simulink model "acquire_data_ag"  (R2017b)
settings: Solver=FixedStepDiscrete  StartTime=0.0  StopTime=10.0  RelTol=1e-3
undefined symbols (not defined in the file or in its folder): RGBLED_COLOR_ENUM, RGBLED_MODE_ENUM
libraries: pixhawk_slib_sensors_actuators x3
settings Model: Creator=Mr Wang  LastModifiedBy=dream
settings OptimizationCC: DefaultParameterBehavior=Inlined  MaxStackSize=128
settings DebuggingCC: ParameterTunabilityLossMsg=error
settings HardwareCC: ProdBitPerPointer=32  ProdBitPerSizeT=32  ProdBitPerPtrDiffT=32  ProdLargestAtomicInteger=Long  ProdLargestAtomicFloat=Double  ProdWordSize=32  ProdHWDeviceType=ARM Compatible->ARM Cortex
settings SFSimCC: MATLABDynamicMemAlloc=off
settings RTWCC: SystemTargetFile=ert.tlc  HardwareBoard=Pixhawk PX4  TemplateMakefile=ert_default_tmf  GenerateReport=on  Toolchain=Pixhawk Toolchain  IncludeHyperlinkInReport=on  LaunchReport=on  GenerateTraceInfo=on  GenerateTraceReport=on  GenerateTraceReportSl=on  GenerateTraceReportSf=on  GenerateTraceReportEml=on
settings CodeAppCC: ForceParamTrailComments=on  IgnoreCustomStorageClasses=off  OperatorAnnotations=on  SimulinkDataObjDesc=on  SFDataObjDesc=on  MATLABFcnDesc=on  InsertBlockDesc=on  StateflowObjectComments=on  MATLABSourceComments=on
settings ERTTargetCC: MultiwordLength=2048  ERTCustomFileTemplate=PX4_codertarget_file_process.tlc

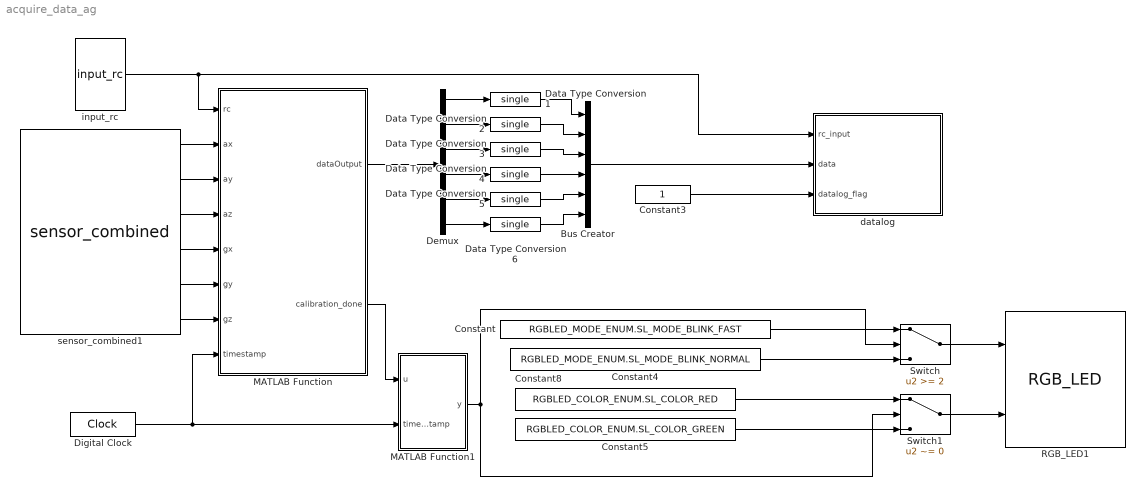
== system acquire_data_ag ==
  Bus Creator : BusCreator  Inputs=6
  Constant : Constant  Value=RGBLED_MODE_ENUM.SL_MODE_BLINK_FAST  OutDataTypeStr=Enum: RGBLED_MODE_ENUM
  Constant3 : Constant  OutDataTypeStr=double
  Constant4 : Constant  Value=RGBLED_MODE_ENUM.SL_MODE_BLINK_NORMAL  OutDataTypeStr=Enum: RGBLED_MODE_ENUM
  Constant5 : Constant  Value=RGBLED_COLOR_ENUM.SL_COLOR_GREEN  OutDataTypeStr=Enum: RGBLED_COLOR_ENUM
  Constant8 : Constant  Value=RGBLED_COLOR_ENUM.SL_COLOR_RED  OutDataTypeStr=Enum: RGBLED_COLOR_ENUM
  Data Type Conversion{1..6} (6 alike) : DataTypeConversion  OutDataTypeStr=single
  Demux : Demux  Outputs=6
  Digital Clock : DigitalClock
  MATLAB Function : MATLAB Function  TreatAsAtomicUnit=on
  MATLAB Function1 : MATLAB Function  TreatAsAtomicUnit=on
  RGB_LED1 : pixhawk_slib_sensors_actuators/RGB_LED  Description=|
      | This block gives the user control over various lighting modes of the RGB LED available on the PX4 hardware. 
      | This block accepts 2 inputs: Mode and Color.  These are enumeration data types.  You can find out what values are valid in the MATLAB command window by typing: 
      | Enumeration members for class 'RGBLED_COLOR_ENUM':
      |     SL_COLOR_OFF
      |     SL_COLOR_RED
      |     SL_COLOR_GREEN
      |     SL_COLOR_BLUE
      |     SL_COLOR_YELLOW
      |     SL_COLOR_PURPLE
      |     SL_COLOR_AMBER
      |     SL_COLOR_CYAN
      |     SL_COLOR_WHITE 
      | Enumeration members for class 'RGBLED_MODE_ENUM':
      |     SL_MODE_OFF
      |     SL_MODE_ON
      |     SL_MODE_DISABLED
      |     SL_MODE_BLINK_SLOW
      |     SL_MODE_BLINK_NORMAL
      |     SL_MODE_BLINK_FAST
      |     SL_MODE_BREATHE  
      | Look at the sample Simulink model: px4demo_rgbled.slx for an example of how to use this block.
      settings: SourceProductName=Pixhawk Target Blocks
  Switch : Switch  Threshold=2
  Switch1 : Switch  Criteria=u2 ~= 0  Threshold=1500
  datalog : Subsystem
  input_rc : pixhawk_slib_sensors_actuators/input_rc  sampletime=1/250  channel1=off  channel2=off  channel3=off  channel4=off  channel5=on  channel6=off  channel7=off  channel8=off  channel9=off  channel10=off  channel11=off  channel12=off  channel13=off  channel14=off  channel15=off  channel16=off  channel17=off  channel18=off  ch_count=off  rssi=off  rc_failsafe=off  rc_lost=off  rc_inputsource=off
      settings: SourceProductName=Pixhawk Target Blocks
  sensor_combined1 : pixhawk_slib_sensors_actuators/sensor_combined  Description=|  sampletime=1/250  show_mag=off  show_acc=on  show_gyro=on  show_baro=off  show_ts=off
      | Sensor Combined Block
      | 
      | This block enables access to the various sensors available on the px4fmu-v2 hardware.  
      | The user can use these signals in the Simulink control model.  
      | The sample time needs to be provided in the mask dialog.  
      | Optional output ports can also be selected.  
      | Refer to the sample model: px4demo_attitude_control.slx
      | 
      | Signal definitions: 
      | Magnetometer (x,y,z) - single values – Magnetic field in NED body frame, in Gauss 
      | Accelerometer (x,y,z) - single values – Acceleration in NED body frame, in m/s^2 
      | Gyroscope (p,q,r) - single values – Angular velocity in radians per second 
      | Barometer (Altitude) - single value – Barometric pressure, already temperature compensated (millibars) 
      | RunTime (timestamp) - double value – Timestamp in microseconds since boot, from gyro 
      |   
      | The sensor_combined block needs to have the px4io service running on the PX4 hardware in order to get valid signal values.
      settings: SourceProductName=Pixhawk Target Blocks
  wires:
  input_rc/1 -> datalog/1(rc_input), MATLAB Function/1(rc)
  Data Type Conversion1/1 -> Bus Creator/1
  Data Type Conversion2/1 -> Bus Creator/2
  Data Type Conversion3/1 -> Bus Creator/3
  Bus Creator/1 -> datalog/2(data)
  MATLAB Function/1(dataOutput) -> Demux/1
  Demux/2 -> Data Type Conversion2/1
  MATLAB Function/2(calibration_done) -> MATLAB Function1/1(u)
  Constant/1 -> Switch/1
  Constant4/1 -> Switch/3
  Switch/1 -> RGB_LED1/1
  Switch1/1 -> RGB_LED1/2
  Constant8/1 -> Switch1/1
  Constant5/1 -> Switch1/3
  Demux/1 -> Data Type Conversion1/1
  Demux/3 -> Data Type Conversion3/1
  Constant3/1 -> datalog/3(datalog_flag)
  Demux/6 -> Data Type Conversion6/1
  Data Type Conversion6/1 -> Bus Creator/6
  Demux/5 -> Data Type Conversion5/1
  Data Type Conversion5/1 -> Bus Creator/5
  Demux/4 -> Data Type Conversion4/1
  Data Type Conversion4/1 -> Bus Creator/4
  Digital Clock/1 -> MATLAB Function/8(timestamp), MATLAB Function1/2(timestamp)
  MATLAB Function1/1(y) -> Switch1/2, Switch/2
  sensor_combined1/1 -> MATLAB Function/2(ax)
  sensor_combined1/2 -> MATLAB Function/3(ay)
  sensor_combined1/3 -> MATLAB Function/4(az)
  sensor_combined1/4 -> MATLAB Function/5(gx)
  sensor_combined1/5 -> MATLAB Function/6(gy)
  sensor_combined1/6 -> MATLAB Function/7(gz)

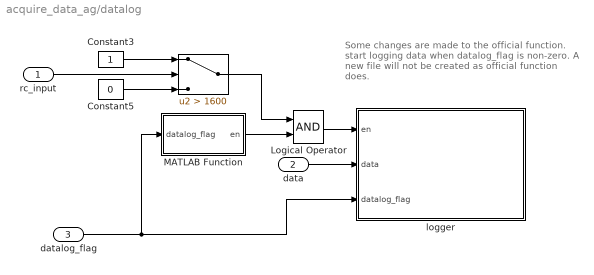
== system acquire_data_ag/datalog ==
  note: Some changes are made to the official
      | function. start logging data when
      | datalog_flag is non-zero. A new file will
      | not be created as official function does.
  rc_input : Inport
  data : Inport  Port=2
  datalog_flag : Inport  Port=3
  " " : Switch  Criteria=u2 > Threshold  Threshold=1600
  Constant3 : Constant
  Constant5 : Constant  Value=0
  Logical Operator : Logic  AllPortsSameDT=off  OutDataTypeStr=boolean
  MATLAB Function : MATLAB Function  TreatAsAtomicUnit=on
  logger : Subsystem  mask(Binary Logger){logfile=/fs/microsd/log/e_acc, cacheflag=off, numRecs=60000}
      mask prompts: cacheflag "Cache in Memory"; numRecs "Max Record Count"
      mask help:
      | Log a vector of data to a file on the SD card
      |
      | If Cache in Memory is on data is written when en goes low or when max number of records specified is reached.
      | Otherwise Max Number of Records is used to indicate when to performa an fflush out to file.
      mask init:
      | logname=uint8(logfile);
      mask Help: eval('pixhawk.internal.doc(''binary_logger_Block.html'')');
      mask Display:
      | fprintf(get_param(gcb,'logfile'))
      | port_label('input',1,'en')
      | port_label('input',2,'data')
      | port_label('input',3,'datalog_flag')
  wires:
  rc_input/1 -> " "/2
  data/1 -> logger/2(data)
  datalog_flag/1 -> logger/3(datalog_flag), MATLAB Function/1(datalog_flag)
  Constant3/1 -> " "/1
  Constant5/1 -> " "/3
  " "/1 -> Logical Operator/1
  MATLAB Function/1(en) -> Logical Operator/2
  Logical Operator/1 -> logger/1(en)

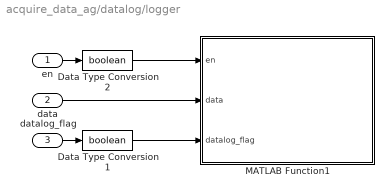
== system acquire_data_ag/datalog/logger ==
  en : Inport
  data : Inport  Port=2
  datalog_flag : Inport  Port=3
  Data Type Conversion1 : DataTypeConversion  OutDataTypeStr=boolean
  Data Type Conversion2 : DataTypeConversion  OutDataTypeStr=boolean
  MATLAB Function1 : MATLAB Function  TreatAsAtomicUnit=on
  wires:
  data/1 -> MATLAB Function1/2(data)
  Data Type Conversion2/1 -> MATLAB Function1/1(en)
  en/1 -> Data Type Conversion2/1
  datalog_flag/1 -> Data Type Conversion1/1
  Data Type Conversion1/1 -> MATLAB Function1/3(datalog_flag)

== matlab function acquire_data_ag/datalog/logger/MATLAB Function1 ==
  data: en input boolean; data input; datalog_flag input boolean; logname parameter uint8; cacheflag parameter boolean; numRecs parameter uint32
%% Binary Logger
% Note: All data needs to be of the same type (e.g. double)
% Header information format:
%           String "MWLOGV##"
%           Time/Date 4 bytes (time())
%           Number of Signals per record Logged 1 byte (256 max)
%           Data Type of Signals Logged  1 byte (1-10)
%           Number of bytes per record 2 bytes (65535 max)
% This does NOT include the number of data sets logged.  
% i.e. The Reader is responsible for reading until EOF.
% MathWorks Pilot Engineering 2015
% Steve Kuznicki
function binary_logger(en, data, datalog_flag, logname, cacheflag, numRecs)
%#codegen
    persistent fp isflushed isopen count lognumstr elem_size vect_size
    coder.cinclude('<stdio.h>');
    coder.cinclude('<time.h>');
    
    if isempty(count)
        count = uint32(0);
        lognumstr = 65;
        isopen = false;
        fp = coder.opaque('FILE*', 'NULL');
        isflushed = false;
        elem_size = uint16(1);
        vect_size = coder.const(uint8(numel(data)));
        if cacheflag == true
            %datastored = zeros(numRecs*uint32(coder.const(numel(data))), 1, 'like', data);
        end
    end

    if (en)
        if isopen == false
            [elsize, eltype] = get_elem_size(data);
            elem_size = coder.const(uint16(elsize));
            elem_type = coder.const(uint8(eltype));
            vect_size = coder.const(uint8(numel(data)));
            coder.ceval('printf',['OPENING file %s vect_size %d elem_size %d numRecs %d %c' uint8(0)], ...
                [logname, '_', char(lognumstr), '.bin', int8(0)], uint32(vect_size), uint32(elem_size), uint32(numRecs), uint8(10));
            fp = coder.ceval('fopen', [logname, '_', char(lognumstr), '.bin', int8(0)], ['wb', int8(0)]);
            lognumstr = lognumstr + 1;
            isflushed = false;
            count = uint32(0);
            isopen = true;
            % Write header information here
            % header token + version
            mlStrVer = 'MWLOGV01';
            coder.ceval('fwrite', coder.rref(mlStrVer), uint32(1), length(mlStrVer), fp);
            % date/time
            tm = uint32(0);
            tmptr = uint32(0);
            tm = coder.ceval('time',coder.wref(tmptr));
            coder.ceval('fwrite', coder.rref(tm), uint32(4), uint32(1), fp);
            % number of elements in each record
            coder.ceval('fwrite', coder.rref(vect_size), uint32(1), uint32(1), fp);
            % data type of the elements
            coder.ceval('fwrite', coder.rref(elem_type), uint32(1), uint32(1), fp);
            % size of each record in bytes
            recSize = elem_size * uint16(vect_size);
            coder.ceval('fwrite', coder.rref(recSize), uint32(2), uint32(1), fp);
        end
        % cache data in memory or use fwrite
        if cacheflag == true
            addr = (count*uint32(vect_size))+1;
            for idx = 1:vect_size
                %datastored(addr) = data(idx);
                addr = addr + 1;
            end
            count = count + uint32(1);
        else
            if  datalog_flag
                coder.ceval('fwrite', coder.rref(data), elem_size, vect_size, fp);
                count = count + uint32(1);
            end
        end
        
        % check for data count limit
        if count >= numRecs
            if cacheflag
                for idx = 1:count*uint32(vect_size)
                    %coder.ceval('fwrite', coder.rref(datastored(idx)), elem_size, uint32(1), fp);
                end
            end
            coder.ceval('fflush', fp);
            isflushed = false;
            count = uint32(0);
        end
    else
        if isopen == true
            if ~isflushed 
                coder.ceval('printf',['CLOSING file. count = %d %c' uint8(0)], uint32(count), uint8(10));
                if cacheflag
                    count = count + uint32(1);
                    for idx = 1:count*uint32(vect_size)
                        %coder.ceval('fwrite', coder.rref(datastored(idx)), elem_size, uint32(1), fp);
                    end
                end
                coder.ceval('fflush', fp);
                isflushed = true;
            end
            coder.ceval('fclose', fp);
        end
        isopen = false;
        count = uint32(0);
    end
end

% return the size of the element in bytes
function [elem_size, dtype] = get_elem_size(data)
    switch(class(data))
        case 'double'
            elem_size = 8;
            dtype = 1;
        case 'single'
            elem_size = 4;
            dtype = 2;
        case 'int32'
            elem_size = 4;
            dtype = 3;
        case 'uint32'
            elem_size = 4;
            dtype = 4;
        case 'int16'
            elem_size = 2;
            dtype = 5;
        case 'uint16'
            elem_size = 2;
            dtype = 6;
        case 'int8'
            elem_size = 1;
            dtype = 7;
        case 'uint8'
            elem_size = 1;
            dtype = 8;
        case 'logical'
            elem_size = 1;
            dtype = 9;
        case 'embedded.fi'
            nt = numerictype(data);
            elem_size = 2^ceil(log2(ceil(nt.WordLength / 8)));
            dtype = 10;
    end
    if ~isreal(data)
        elem_size = elem_size*2;
    end
    
    elem_size = uint16(elem_size);
    dtype = uint8(dtype);
end

== matlab function acquire_data_ag/MATLAB Function ==
  data: rc input; ax input; ay input; az input; gx input; gy input; gz input; timestamp input; dataOutput output single; calibration_done output double
function [dataOutput, calibration_done]  = fcn(rc, ax, ay, az, gx, gy, gz, timestamp)
%Function description:
%  Collect data for accelerometer calibration. The collected data includes
%  the feature points and all accelerometer data after the data logging is
%  enabled. The principle of selecting feature points is that the variance
%  of consecutive _onceSample_ points is smaller than _std_acc_, and the
%  distance from all previous feature points is greater than _mindist_.
%Input:
%  rc: the remote control input, in the range of 1000-2000, and when rc >
%       1600, start collecting data. 
%  ax, ay, az, gx, gy, gz: the value of the accelerometer and gyroscope read
%                                from the IMU, in m/s2, rad/s respectively. 
%  timestamp: timestamp, in seconds
%Output:
%  dataOutput: 6-dimensional array, the first three are the values of the
%                     accelerometer; the last three are feature points.
%  calibration_done：If a feature point is collected calibration_done =1,
%                               else calibration_done = 0.

    g = 9.8;  %  gravitational acceleration
    onceSample = 100;  %  single sample number for averaging
    sample_max_points = 10;  %  number of feature points required
    mindist = 0.1*g;  %  minimum distance between two feature points
    std_acc = 0.005*g; 
    persistent accData;
    if  isempty(accData)
        accData = single(zeros(onceSample, 3));
    end
    persistent acc_valid;
    if  isempty(acc_valid)
        acc_valid = single(zeros(sample_max_points, 3));
    end
     persistent samplecount;
    if  isempty(samplecount)
        samplecount = 1;
    end
    persistent vcount;
    if  isempty(vcount)
        vcount = 0;
    end
    persistent log_finished;
    if  isempty(log_finished)
        log_finished = false;
    end
 
    acc_average = single(zeros(1, 3));
    dataOutput = single(zeros(6, 1));
    if rc > 1600 && ~log_finished  % manually control whether to log data
        if detect_state(timestamp, gx, gy, gz)  %  check if the board is rotating
            accData(samplecount, :) = single([ax, ay, az]);
            samplecount = samplecount + 1;
        else
              samplecount = 1;
        end
        if samplecount > onceSample  
            %  The number of single sampled data reaches the specified
            %  value, and average the data as an alternative feature point.
            samplecount = 1;
            accData1 = zeros(onceSample, 1);
            for i = 1:onceSample
                accData1(i) = norm(accData(i, :));
            end
            if std(accData1) < std_acc   
                 acc_average = mean(accData, 1);
                 acc_valid_flag = true;
               
                 if vcount ~= 0
                     for k = 1 : vcount  
                         dis = norm(acc_average - acc_valid(k, 1:3));
                         if dis < mindist  
                             %  discard the alternative feature point if the distance is too small
                            acc_valid_flag = false;
                            break;
                         end
                     end
                     if acc_valid_flag
                        vcount = vcount + 1;  %  the number of collected feature points
                        acc_valid(vcount, 1:3) = acc_average;  %  record the feature point
                     end
                else
                    vcount = 1;  %  first sampling
                    acc_valid(vcount, 1:3) = acc_average;
                 end
            else
                %The collected accelerometer data is noisy and start to collect data again.
                samplecount = 1;
                acc_valid_flag = false;
            end
        else
            acc_valid_flag = false;
        end
    else
        acc_valid_flag = false;
    end
     if ~acc_valid_flag
         dataOutput = [ax, ay, az, 0, 0, 0]';
         calibration_done = 0;
     else
         dataOutput(1:3) = [ax, ay, az]';
         dataOutput(4:6) = acc_average';
         calibration_done = 1;
     end
    if vcount >= sample_max_points  
        %The number of feature points meet the requirement.
        log_finished = true;
    else
        log_finished = false;
    end
end
    
function isStable = detect_state(timestamp, gx, gy, gz)
 %Function description:
%  The gyroscope data is used to detect whether the board is rotating. The
%  2-norm of gyroscope  is less than 0.1 for one second, that is, the board
%  is considered to be stationary.
%Input:
%  timestamp: unit:s
%  gx, gy, gz: gyroscope data, unit: rad/s
%Output:
%  isStable: if the board is stationary, isStable = true ,else isStable = false.

    persistent t;
    if  isempty(t)
        t = timestamp;
    end
    persistent flag;
    if  isempty(flag)
        flag = 0;
    end
    
    if norm([gx, gy, gz]) < 0.1 && flag < 0.5
        t = timestamp;
        flag = 1;
    end
    if norm([gx, gy, gz]) > 0.1
        flag = 0;
        t = timestamp;
    end
    if timestamp - t > 1
        isStable = true;
    else
        isStable = false;
    end
end

== matlab function acquire_data_ag/datalog/MATLAB Function ==
  data: datalog_flag input; en output
function en = fcn(datalog_flag)

persistent count;
if isempty(count)
    count=0;
end

if datalog_flag
    count=count+1;
end
if count > 60000
    en = false;
    count = 0;
else
    en = true;
end

== matlab function acquire_data_ag/MATLAB Function1 ==
  data: u input; y output; timestamp input
function y = fcn(u, timestamp)
 %Function description:
%  Control LED lights to indicate whether data collection is complete.
%Input:
%  u: Whether valid accelerometer data is collected. u = 0, indicating that it has not been acquired; u = 1, indicating that valid data has been collected.
%  timestamp: uint:s.
%Output:
%  y: No feature point is collected, y = 0; one feature point is collected, y = 1; 10 feature point are collected, y = 2.
    persistent t;
    if  isempty(t)
        t = timestamp;
    end
    persistent led_t;
    if  isempty(led_t)
        led_t = 0;
    end
    persistent a_count;
    if  isempty(a_count)
        a_count = 0;
    end
    if u > 0.5 
        led_t = 1;
        t = timestamp;
        a_count = a_count + 1;
    end
        
    if led_t > 0.5 && timestamp - t < 3
        y = 1;
        if a_count > 9
            y = 2;
        end
    else
        y = 0;
        led_t = 0;
    end
end
